simulink model "GaitAlgorithm_arduino_V3_2023a"  (R2023a)
settings: Solver=FixedStepAuto  StartTime=0.0  StopTime=inf  RelTol=1e-3  EnableMultiTasking=on
undefined symbols (not defined in the file): DiscIntNeverNeededParam, f
libraries: simulink x16, mcp2515lib x13, matrix_library x6, arduinosensorlib x4, eeGeneralControl x4, arduinolib x2, instrumentlib x2
(part 2 of 2)

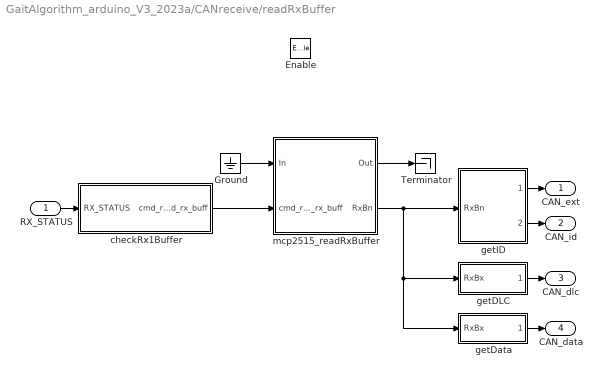
== system GaitAlgorithm_arduino_V3_2023a/CANreceive/readRxBuffer ==
  RX_STATUS : Inport
  Enable : EnablePort
  Ground : Ground
  Terminator : Terminator
  checkRx1Buffer : Subsystem  TreatAsAtomicUnit=on
  getDLC : Subsystem  TreatAsAtomicUnit=on
  getData : Subsystem  TreatAsAtomicUnit=on
  getID : Subsystem  TreatAsAtomicUnit=on
      settings: RTWSystemCode=Inline
  mcp2515_readRxBuffer : Subsystem  TreatAsAtomicUnit=on
  CAN_ext : Outport
  CAN_id : Outport  Port=2
  CAN_dlc : Outport  Port=3
  CAN_data : Outport  Port=4
  wires:
  getData/1(CAN_data) -> CAN_data/1
  mcp2515_readRxBuffer/2(RxBn) -> getID/1(RxBn), getData/1(RxBx), getDLC/1(RxBx)
  getID/2(CAN_id) -> CAN_id/1
  getID/1(CAN_ext) -> CAN_ext/1
  getDLC/1(CAN_dlc) -> CAN_dlc/1
  mcp2515_readRxBuffer/1(Out) -> Terminator/1
  Ground/1 -> mcp2515_readRxBuffer/1(In)
  RX_STATUS/1 -> checkRx1Buffer/1(RX_STATUS)
  checkRx1Buffer/1(cmd_read_rx_buff) -> mcp2515_readRxBuffer/2(cmd_read_rx_buff)

== system GaitAlgorithm_arduino_V3_2023a/CANtransmit/check TxB0 ==
  In1 : Inport
  Bitmask_TxReq : simulink/Logic and Bit Operations/Bitwise Operator  logicop=AND  UseBitMask=on  BitMask=bin2dec('00001000')  BitMaskRealWorld=Stored Integer
  CAN_FAIL : Constant  Value=2  OutDataTypeStr=int8
  CAN_OK : Constant  OutDataTypeStr=int8
  MCP_TxB0CTRL1 : Constant  Value=hex2dec('30')  OutDataTypeStr=uint8
  Switch : Switch  Criteria=u2 > Threshold  SaturateOnIntegerOverflow=off  InputSameDT=off
  mcp2515_readRegister : Subsystem  TreatAsAtomicUnit=on
  Out1 : Outport
  CANTx_Transmit : Outport  Port=2
  wires:
  CAN_FAIL/1 -> Switch/3
  mcp2515_readRegister/1(Out) -> Out1/1
  mcp2515_readRegister/2(SPI_data) -> Bitmask_TxReq/1
  MCP_TxB0CTRL1/1 -> mcp2515_readRegister/2(address)
  Bitmask_TxReq/1 -> Switch/2
  Switch/1 -> CANTx_Transmit/1
  CAN_OK/1 -> Switch/1
  In1/1 -> mcp2515_readRegister/1(In)

== system GaitAlgorithm_arduino_V3_2023a/CANtransmit/load Tx data ==
  In1 : Inport
  CAN_ext : Inport  Port=2
  CAN_id : Inport  Port=3
  CAN_dlc : Inport  Port=4
  CAN_data : Inport  Port=5
  MCP_load_TxB0 : Constant  Value=hex2dec('40')  OutDataTypeStr=uint8
  Vector Concatenate : Concatenate  NumInputs=3
  mcp2515_writeTxBuffer : Subsystem  TreatAsAtomicUnit=on
  setID : Subsystem  TreatAsAtomicUnit=on
      settings: RTWSystemCode=Inline
  Out1 : Outport
  wires:
  CAN_ext/1 -> setID/1(ext)
  CAN_id/1 -> setID/2(id)
  CAN_data/1 -> Vector Concatenate/3
  CAN_dlc/1 -> Vector Concatenate/2
  setID/1(TxBn_ID) -> Vector Concatenate/1
  In1/1 -> mcp2515_writeTxBuffer/1(In)
  mcp2515_writeTxBuffer/1(Out) -> Out1/1
  MCP_load_TxB0/1 -> mcp2515_writeTxBuffer/2(cmd_load_tx_buff)
  Vector Concatenate/1 -> mcp2515_writeTxBuffer/3(data_tx_buff)

== system GaitAlgorithm_arduino_V3_2023a/CANtransmit/send TxB0 ==
  In1 : Inport
  MCP_TxB0CTRL : Constant  Value=hex2dec('30')  OutDataTypeStr=uint8
  TxREQ : Constant  Value=8  OutDataTypeStr=uint8
  mcp2515_writeRegister : Subsystem  TreatAsAtomicUnit=on
  Out1 : Outport
  wires:
  MCP_TxB0CTRL/1 -> mcp2515_writeRegister/2(address)
  mcp2515_writeRegister/1(Out) -> Out1/1
  In1/1 -> mcp2515_writeRegister/1(In)
  TxREQ/1 -> mcp2515_writeRegister/3(value)

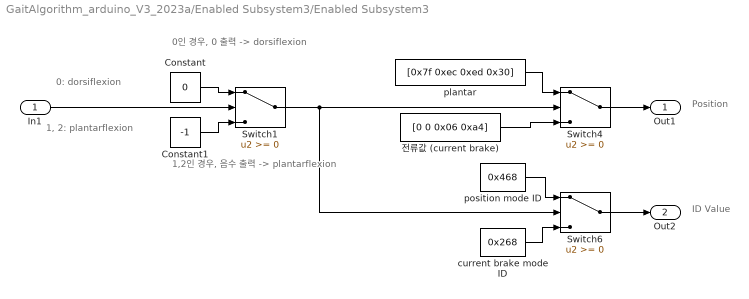
== system GaitAlgorithm_arduino_V3_2023a/Enabled Subsystem3/Enabled Subsystem3 ==
  note: ID Value
  note: Position
  note: 1,2인 경우, 음수 출력 -> plantarflexion
  note: 0인 경우, 0 출력 -> dorsiflexion
  note: 1, 2: plantarflexion
  note: 0: dorsiflexion
  In1 : Inport
  Constant : Constant  Value=0
  Constant1 : Constant  Value=-1
  Switch1 : Switch  SaturateOnIntegerOverflow=off  InputSameDT=off
  Switch4 : Switch  OutDataTypeStr=uint32  SaturateOnIntegerOverflow=off  InputSameDT=off
  Switch6 : Switch  OutDataTypeStr=uint32  SaturateOnIntegerOverflow=off  InputSameDT=off
  current brake mode ID : Constant  Value=0x268
  plantar : Constant  Value=[0x7f 0xec 0xed 0x30]
  position mode ID : Constant  Value=0x468
  전류값 (current brake) : Constant  Value=[0 0 0x06 0xa4]  OutDataTypeStr=uint8
  Out1 : Outport
  Out2 : Outport  Port=2
  wires:
  Switch6/1 -> Out2/1
  plantar/1 -> Switch4/1
  전류값 (current brake)/1 -> Switch4/3
  position mode ID/1 -> Switch6/1
  current brake mode ID/1 -> Switch6/3
  Switch4/1 -> Out1/1
  In1/1 -> Switch1/2
  Constant/1 -> Switch1/1
  Constant1/1 -> Switch1/3
  Switch1/1 -> Switch6/2, Switch4/2

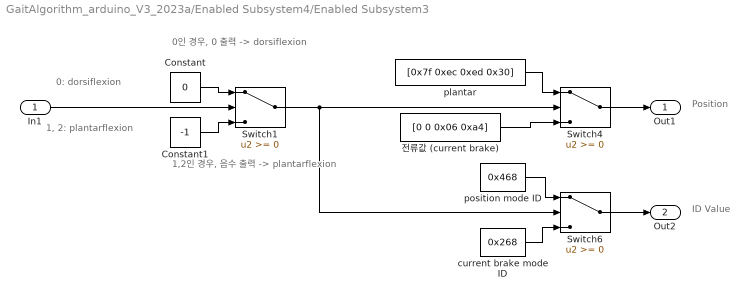
== system GaitAlgorithm_arduino_V3_2023a/Enabled Subsystem4/Enabled Subsystem3 ==
  note: ID Value
  note: Position
  note: 1,2인 경우, 음수 출력 -> plantarflexion
  note: 0인 경우, 0 출력 -> dorsiflexion
  note: 1, 2: plantarflexion
  note: 0: dorsiflexion
  In1 : Inport
  Constant : Constant  Value=0
  Constant1 : Constant  Value=-1
  Switch1 : Switch  SaturateOnIntegerOverflow=off  InputSameDT=off
  Switch4 : Switch  OutDataTypeStr=uint32  SaturateOnIntegerOverflow=off  InputSameDT=off
  Switch6 : Switch  OutDataTypeStr=uint32  SaturateOnIntegerOverflow=off  InputSameDT=off
  current brake mode ID : Constant  Value=0x268
  plantar : Constant  Value=[0x7f 0xec 0xed 0x30]
  position mode ID : Constant  Value=0x468
  전류값 (current brake) : Constant  Value=[0 0 0x06 0xa4]  OutDataTypeStr=uint8
  Out1 : Outport
  Out2 : Outport  Port=2
  wires:
  Switch6/1 -> Out2/1
  plantar/1 -> Switch4/1
  전류값 (current brake)/1 -> Switch4/3
  position mode ID/1 -> Switch6/1
  current brake mode ID/1 -> Switch6/3
  Switch4/1 -> Out1/1
  In1/1 -> Switch1/2
  Constant/1 -> Switch1/1
  Constant1/1 -> Switch1/3
  Switch1/1 -> Switch6/2, Switch4/2

== system GaitAlgorithm_arduino_V3_2023a/CANbegin/setup/changeCANmode(config) ==
  In : Inport
  MCP_CANCTRL : Constant  Value=hex2dec('0F')  OutDataTypeStr=uint8
  MODE_CONFIG : Constant  Value=hex2dec('80')  OutDataTypeStr=uint8
  MODE_MASK : Constant  Value=hex2dec('E0')  OutDataTypeStr=uint8
  mcp2515_modifyRegister : Subsystem  TreatAsAtomicUnit=on
  Out : Outport
  wires:
  MODE_CONFIG/1 -> mcp2515_modifyRegister/4(data)
  MODE_MASK/1 -> mcp2515_modifyRegister/3(mask)
  MCP_CANCTRL/1 -> mcp2515_modifyRegister/2(address)
  In/1 -> mcp2515_modifyRegister/1(In)
  mcp2515_modifyRegister/1(Out) -> Out/1

== system GaitAlgorithm_arduino_V3_2023a/CANbegin/setup/changeCANmode(normal) ==
  In : Inport
  MCP_CANCTRL : Constant  Value=hex2dec('0F')  OutDataTypeStr=uint8
  MODE_MASK : Constant  Value=hex2dec('E0')  OutDataTypeStr=uint8
  MODE_NORMAL : Constant  Value=0  OutDataTypeStr=uint8
  mcp2515_modifyRegister : Subsystem  TreatAsAtomicUnit=on
  Out : Outport
  wires:
  MODE_MASK/1 -> mcp2515_modifyRegister/3(mask)
  MODE_NORMAL/1 -> mcp2515_modifyRegister/4(data)
  MCP_CANCTRL/1 -> mcp2515_modifyRegister/2(address)
  In/1 -> mcp2515_modifyRegister/1(In)
  mcp2515_modifyRegister/1(Out) -> Out/1

== system GaitAlgorithm_arduino_V3_2023a/CANbegin/setup/mcp2515_reset ==
  In : Inport
  MCP_RESET : Constant  Value=hex2dec('C0')  OutDataTypeStr=uint8
  SPI driver : mcp2515lib/CAN application/mcp2515 driver/SPI driver  SystemSampleTime=-1  VariantActivationTime=update diagram  Latency=0  AutoFrameSizeCalculation=off
      settings: SourceProductName=CAN device driver for mcp2515
  Temporary buffer : DataStoreWrite  DataStoreName=temp_1byte  IndexOptions=Index vector (dialog)  Indices=1  OutputSizes=1
  Out : Outport
  wires:
  MCP_RESET/1 -> SPI driver/1
  In/1 -> Out/1
  SPI driver/1 -> Temporary buffer/1

== system GaitAlgorithm_arduino_V3_2023a/CANbegin/setup/setCANRxBuffer ==
  note: RXB0
  note: RXB1
  note: no filter, no mask
  In : Inport
  MCP_RXB0CTRL : Constant  Value=hex2dec('60')  OutDataTypeStr=uint8
  MCP_RXB1CTRL : Constant  Value=hex2dec('70')  OutDataTypeStr=uint8
  MCP_RXB_RX_MASK : Constant  Value=hex2dec('60')  OutDataTypeStr=uint8
  mcp2515_writeRegister : Subsystem  TreatAsAtomicUnit=on
  mcp2515_writeRegister1 : Subsystem  TreatAsAtomicUnit=on
  Out : Outport
  wires:
  MCP_RXB0CTRL/1 -> mcp2515_writeRegister/2(address)
  MCP_RXB1CTRL/1 -> mcp2515_writeRegister1/2(address)
  MCP_RXB_RX_MASK/1 -> mcp2515_writeRegister1/3(value), mcp2515_writeRegister/3(value)
  In/1 -> mcp2515_writeRegister/1(In)
  mcp2515_writeRegister1/1(Out) -> Out/1
  mcp2515_writeRegister/1(Out) -> mcp2515_writeRegister1/1(In)

== system GaitAlgorithm_arduino_V3_2023a/CANbegin/setup/setCANspeed ==
  In : Inport
  CNF1 : Inport  Port=2
  CNF2 : Inport  Port=3
  CNF3 : Inport  Port=4
  MCP_CNF1 : Constant  Value=hex2dec('2A')  OutDataTypeStr=uint8
  MCP_CNF2 : Constant  Value=hex2dec('29')  OutDataTypeStr=uint8
  MCP_CNF3 : Constant  Value=hex2dec('28')  OutDataTypeStr=uint8
  mcp2515_writeRegister1 : Subsystem  TreatAsAtomicUnit=on
  mcp2515_writeRegister2 : Subsystem  TreatAsAtomicUnit=on
  mcp2515_writeRegister3 : Subsystem  TreatAsAtomicUnit=on
  Out : Outport
  wires:
  MCP_CNF2/1 -> mcp2515_writeRegister2/2(address)
  MCP_CNF3/1 -> mcp2515_writeRegister3/2(address)
  CNF3/1 -> mcp2515_writeRegister3/3(value)
  CNF1/1 -> mcp2515_writeRegister1/3(value)
  MCP_CNF1/1 -> mcp2515_writeRegister1/2(address)
  CNF2/1 -> mcp2515_writeRegister2/3(value)
  In/1 -> mcp2515_writeRegister1/1(In)
  mcp2515_writeRegister1/1(Out) -> mcp2515_writeRegister2/1(In)
  mcp2515_writeRegister2/1(Out) -> mcp2515_writeRegister3/1(In)
  mcp2515_writeRegister3/1(Out) -> Out/1

== system GaitAlgorithm_arduino_V3_2023a/CANreceive/readRxBuffer/checkRx1Buffer ==
  RX_STATUS : Inport
  Bitmask_RxB1_Status : simulink/Logic and Bit Operations/Bitwise Operator  logicop=AND  UseBitMask=on  BitMask=bin2dec('10000000')  BitMaskRealWorld=Stored Integer
  MCP_READ_RxB0 : Constant  Value=hex2dec('90')  OutDataTypeStr=uint8
  MCP_READ_RxB1 : Constant  Value=hex2dec('94')  OutDataTypeStr=uint8
  Switch : Switch  Criteria=u2 > Threshold  SaturateOnIntegerOverflow=off  InputSameDT=off
  cmd_read_rx_buff : Outport
  wires:
  Switch/1 -> cmd_read_rx_buff/1
  MCP_READ_RxB1/1 -> Switch/1
  MCP_READ_RxB0/1 -> Switch/3
  Bitmask_RxB1_Status/1 -> Switch/2
  RX_STATUS/1 -> Bitmask_RxB1_Status/1

== system GaitAlgorithm_arduino_V3_2023a/CANreceive/readRxBuffer/getDLC ==
  RxBx : Inport
  Bitwise Operator : simulink/Logic and Bit Operations/Bitwise Operator  logicop=AND  UseBitMask=off  NumInputPorts=2  BitMask=bin2dec('11011001')  BitMaskRealWorld=Stored Integer
  MCP_DLC_MASK : Constant  Value=hex2dec('0F')  OutDataTypeStr=uint8
  RxDLC : Selector  IndexMode=Zero-based  InputPortWidth=13  IndexOptions=Index vector (dialog)  Indices=4  OutputSizes=1
  CAN_dlc : Outport
  wires:
  Bitwise Operator/1 -> CAN_dlc/1
  RxBx/1 -> RxDLC/1
  RxDLC/1 -> Bitwise Operator/1
  MCP_DLC_MASK/1 -> Bitwise Operator/2

== system GaitAlgorithm_arduino_V3_2023a/CANreceive/readRxBuffer/getData ==
  RxBx : Inport
  RxData : Selector  IndexMode=Zero-based  InputPortWidth=13  IndexOptions=Index vector (dialog)  Indices=[5:12]  OutputSizes=1
  CAN_data : Outport
  wires:
  RxBx/1 -> RxData/1
  RxData/1 -> CAN_data/1

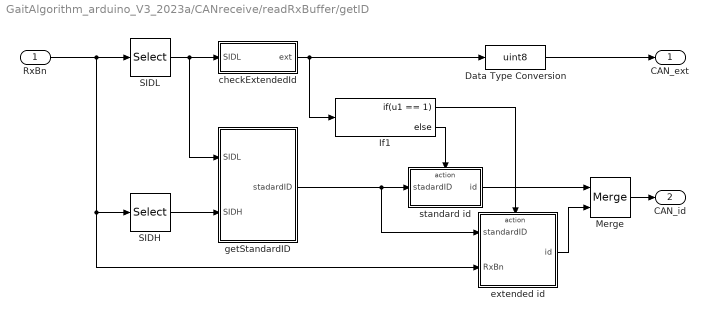
== system GaitAlgorithm_arduino_V3_2023a/CANreceive/readRxBuffer/getID ==
  RxBn : Inport
  Data Type Conversion : DataTypeConversion  OutDataTypeStr=uint8  RndMeth=Simplest  SaturateOnIntegerOverflow=off
  If1 : If  IfExpression=u1 == 1
  Merge : Merge
  SIDH : Selector  IndexMode=Zero-based  InputPortWidth=13  IndexOptions=Index vector (dialog)  Indices=0  OutputSizes=1
  SIDL : Selector  IndexMode=Zero-based  InputPortWidth=13  IndexOptions=Index vector (dialog)  Indices=1  OutputSizes=1
  checkExtendedId : Subsystem
  extended id : Subsystem  TreatAsAtomicUnit=on
      settings: RTWSystemCode=Inline
  getStandardID : Subsystem
  standard id : Subsystem  TreatAsAtomicUnit=on
      settings: RTWSystemCode=Inline
  CAN_ext : Outport
  CAN_id : Outport  Port=2
  wires:
  standard id/1(id) -> Merge/1
  extended id/1(id) -> Merge/2
  Merge/1 -> CAN_id/1
  If1/2 -> standard id/Action
  If1/1 -> extended id/Action
  RxBn/1 -> extended id/2(RxBn), SIDH/1, SIDL/1
  getStandardID/1(stadardID) -> standard id/1(stadardID), extended id/1(standardID)
  SIDL/1 -> getStandardID/1(SIDL), checkExtendedId/1(SIDL)
  SIDH/1 -> getStandardID/2(SIDH)
  checkExtendedId/1(ext) -> Data Type Conversion/1, If1/1
  Data Type Conversion/1 -> CAN_ext/1

== system GaitAlgorithm_arduino_V3_2023a/CANreceive/readRxBuffer/mcp2515_readRxBuffer ==
  In : Inport
  cmd_read_rx_buff : Inport  Port=2
  Constant : Constant  Value=zeros(1,13)  OutDataTypeStr=uint8
  SPI driver : mcp2515lib/CAN application/mcp2515 driver/SPI driver  SystemSampleTime=-1  VariantActivationTime=update diagram  Latency=0  AutoFrameSizeCalculation=off
      settings: SourceProductName=CAN device driver for mcp2515
  Selector1 : Selector  IndexMode=Zero-based  InputPortWidth=14  IndexOptions=Index vector (dialog)  Indices=[1:13]  OutputSizes=1
  Vector Concatenate : Concatenate
  Out : Outport
  RxBn : Outport  Port=2
  wires:
  cmd_read_rx_buff/1 -> Vector Concatenate/1
  Constant/1 -> Vector Concatenate/2
  Vector Concatenate/1 -> SPI driver/1
  SPI driver/1 -> Selector1/1
  Selector1/1 -> RxBn/1
  In/1 -> Out/1

== system GaitAlgorithm_arduino_V3_2023a/CANtransmit/check TxB0/mcp2515_readRegister ==
  In : Inport
  address : Inport  Port=2  OutDataTypeStr=uint8
  Constant : Constant  Value=0  OutDataTypeStr=uint8
  MCP_READ : Constant  Value=3  OutDataTypeStr=uint8
  SPI driver : mcp2515lib/CAN application/mcp2515 driver/SPI driver  SystemSampleTime=-1  VariantActivationTime=update diagram  Latency=0  AutoFrameSizeCalculation=off
      settings: SourceProductName=CAN device driver for mcp2515
  Selector : Selector  IndexMode=Zero-based  InputPortWidth=3  IndexOptions=Index vector (dialog)  Indices=2  OutputSizes=1
  Vector Concatenate : Concatenate  NumInputs=3
  Out : Outport
  SPI_data : Outport  Port=2
  wires:
  SPI driver/1 -> Selector/1
  address/1 -> Vector Concatenate/2
  Constant/1 -> Vector Concatenate/3
  In/1 -> Out/1
  MCP_READ/1 -> Vector Concatenate/1
  Selector/1 -> SPI_data/1
  Vector Concatenate/1 -> SPI driver/1

== system GaitAlgorithm_arduino_V3_2023a/CANtransmit/load Tx data/mcp2515_writeTxBuffer ==
  In : Inport
  cmd_load_tx_buff : Inport  Port=2
  data_tx_buff : Inport  Port=3
  SPI driver : mcp2515lib/CAN application/mcp2515 driver/SPI driver  SystemSampleTime=-1  VariantActivationTime=update diagram  Latency=0  AutoFrameSizeCalculation=off
      settings: SourceProductName=CAN device driver for mcp2515
  Selector1 : Selector  IndexMode=Zero-based  InputPortWidth=14  IndexOptions=Index vector (dialog)  Indices=0  OutputSizes=1
  Temporary buffer : DataStoreWrite  DataStoreName=temp_1byte  IndexOptions=Index vector (dialog)  Indices=1  OutputSizes=1
  Vector Concatenate : Concatenate
  Out : Outport
  wires:
  In/1 -> Out/1
  SPI driver/1 -> Selector1/1
  data_tx_buff/1 -> Vector Concatenate/2
  cmd_load_tx_buff/1 -> Vector Concatenate/1
  Selector1/1 -> Temporary buffer/1
  Vector Concatenate/1 -> SPI driver/1

== system GaitAlgorithm_arduino_V3_2023a/CANtransmit/load Tx data/setID ==
  ext : Inport
  id : Inport  Port=2
  Extended ID : Subsystem  TreatAsAtomicUnit=on
  If : If
  Merge : Merge
  Standard ID : Subsystem  TreatAsAtomicUnit=on
  TxBn_ID : Outport
  wires:
  ext/1 -> If/1
  If/1 -> Extended ID/Action
  If/2 -> Standard ID/Action
  Extended ID/1(TxBn_ID) -> Merge/2
  Standard ID/1(TxBn_ID) -> Merge/1
  Merge/1 -> TxBn_ID/1
  id/1 -> Extended ID/1(id), Standard ID/1(id)

== system GaitAlgorithm_arduino_V3_2023a/CANtransmit/send TxB0/mcp2515_writeRegister ==
  In : Inport
  address : Inport  Port=2  OutDataTypeStr=uint8
  value : Inport  Port=3  OutDataTypeStr=uint8
  MCP_WRITE : Constant  Value=2  OutDataTypeStr=uint8
  SPI driver : mcp2515lib/CAN application/mcp2515 driver/SPI driver  SystemSampleTime=-1  VariantActivationTime=update diagram  Latency=0  AutoFrameSizeCalculation=off
      settings: SourceProductName=CAN device driver for mcp2515
  Selector : Selector  IndexMode=Zero-based  InputPortWidth=3  IndexOptions=Index vector (dialog)  Indices=0  OutputSizes=1
  Temporary buffer : DataStoreWrite  DataStoreName=temp_1byte  IndexOptions=Index vector (dialog)  Indices=1  OutputSizes=1
  Vector Concatenate : Concatenate  NumInputs=3
  Out : Outport
  wires:
  SPI driver/1 -> Selector/1
  Selector/1 -> Temporary buffer/1
  In/1 -> Out/1
  Vector Concatenate/1 -> SPI driver/1
  value/1 -> Vector Concatenate/3
  address/1 -> Vector Concatenate/2
  MCP_WRITE/1 -> Vector Concatenate/1

== system GaitAlgorithm_arduino_V3_2023a/CANbegin/setup/changeCANmode(config)/mcp2515_modifyRegister ==
  In : Inport
  address : Inport  Port=2
  mask : Inport  Port=3
  data : Inport  Port=4
  MCP_BITMOD : Constant  Value=5  OutDataTypeStr=uint8
  SPI driver : mcp2515lib/CAN application/mcp2515 driver/SPI driver  SystemSampleTime=-1  VariantActivationTime=update diagram  Latency=0  AutoFrameSizeCalculation=off
      settings: SourceProductName=CAN device driver for mcp2515
  Selector : Selector  IndexMode=Zero-based  InputPortWidth=4  IndexOptions=Index vector (dialog)  Indices=0  OutputSizes=1
  Temporary buffer : DataStoreWrite  DataStoreName=temp_1byte  IndexOptions=Index vector (dialog)  Indices=1  OutputSizes=1
  Vector Concatenate : Concatenate  NumInputs=4
  Out : Outport
  wires:
  SPI driver/1 -> Selector/1
  data/1 -> Vector Concatenate/4
  address/1 -> Vector Concatenate/2
  mask/1 -> Vector Concatenate/3
  MCP_BITMOD/1 -> Vector Concatenate/1
  In/1 -> Out/1
  Selector/1 -> Temporary buffer/1
  Vector Concatenate/1 -> SPI driver/1

== system GaitAlgorithm_arduino_V3_2023a/CANbegin/setup/changeCANmode(normal)/mcp2515_modifyRegister ==
  In : Inport
  address : Inport  Port=2
  mask : Inport  Port=3
  data : Inport  Port=4
  MCP_BITMOD : Constant  Value=5  OutDataTypeStr=uint8
  SPI driver : mcp2515lib/CAN application/mcp2515 driver/SPI driver  SystemSampleTime=-1  VariantActivationTime=update diagram  Latency=0  AutoFrameSizeCalculation=off
      settings: SourceProductName=CAN device driver for mcp2515
  Selector : Selector  IndexMode=Zero-based  InputPortWidth=4  IndexOptions=Index vector (dialog)  Indices=0  OutputSizes=1
  Temporary buffer : DataStoreWrite  DataStoreName=temp_1byte  IndexOptions=Index vector (dialog)  Indices=1  OutputSizes=1
  Vector Concatenate : Concatenate  NumInputs=4
  Out : Outport
  wires:
  SPI driver/1 -> Selector/1
  data/1 -> Vector Concatenate/4
  address/1 -> Vector Concatenate/2
  mask/1 -> Vector Concatenate/3
  MCP_BITMOD/1 -> Vector Concatenate/1
  In/1 -> Out/1
  Selector/1 -> Temporary buffer/1
  Vector Concatenate/1 -> SPI driver/1

== system GaitAlgorithm_arduino_V3_2023a/CANbegin/setup/setCANRxBuffer/mcp2515_writeRegister ==
  In : Inport
  address : Inport  Port=2  OutDataTypeStr=uint8
  value : Inport  Port=3  OutDataTypeStr=uint8
  MCP_WRITE : Constant  Value=2  OutDataTypeStr=uint8
  SPI driver : mcp2515lib/CAN application/mcp2515 driver/SPI driver  SystemSampleTime=-1  VariantActivationTime=update diagram  Latency=0  AutoFrameSizeCalculation=off
      settings: SourceProductName=CAN device driver for mcp2515
  Selector : Selector  IndexMode=Zero-based  InputPortWidth=3  IndexOptions=Index vector (dialog)  Indices=0  OutputSizes=1
  Temporary buffer : DataStoreWrite  DataStoreName=temp_1byte  IndexOptions=Index vector (dialog)  Indices=1  OutputSizes=1
  Vector Concatenate : Concatenate  NumInputs=3
  Out : Outport
  wires:
  SPI driver/1 -> Selector/1
  Selector/1 -> Temporary buffer/1
  In/1 -> Out/1
  Vector Concatenate/1 -> SPI driver/1
  value/1 -> Vector Concatenate/3
  address/1 -> Vector Concatenate/2
  MCP_WRITE/1 -> Vector Concatenate/1

== system GaitAlgorithm_arduino_V3_2023a/CANbegin/setup/setCANRxBuffer/mcp2515_writeRegister1 ==
  In : Inport
  address : Inport  Port=2  OutDataTypeStr=uint8
  value : Inport  Port=3  OutDataTypeStr=uint8
  MCP_WRITE : Constant  Value=2  OutDataTypeStr=uint8
  SPI driver : mcp2515lib/CAN application/mcp2515 driver/SPI driver  SystemSampleTime=-1  VariantActivationTime=update diagram  Latency=0  AutoFrameSizeCalculation=off
      settings: SourceProductName=CAN device driver for mcp2515
  Selector : Selector  IndexMode=Zero-based  InputPortWidth=3  IndexOptions=Index vector (dialog)  Indices=0  OutputSizes=1
  Temporary buffer : DataStoreWrite  DataStoreName=temp_1byte  IndexOptions=Index vector (dialog)  Indices=1  OutputSizes=1
  Vector Concatenate : Concatenate  NumInputs=3
  Out : Outport
  wires:
  SPI driver/1 -> Selector/1
  Selector/1 -> Temporary buffer/1
  In/1 -> Out/1
  Vector Concatenate/1 -> SPI driver/1
  value/1 -> Vector Concatenate/3
  address/1 -> Vector Concatenate/2
  MCP_WRITE/1 -> Vector Concatenate/1

== system GaitAlgorithm_arduino_V3_2023a/CANbegin/setup/setCANspeed/mcp2515_writeRegister1 ==
  In : Inport
  address : Inport  Port=2  OutDataTypeStr=uint8
  value : Inport  Port=3  OutDataTypeStr=uint8
  MCP_WRITE : Constant  Value=2  OutDataTypeStr=uint8
  SPI driver : mcp2515lib/CAN application/mcp2515 driver/SPI driver  SystemSampleTime=-1  VariantActivationTime=update diagram  Latency=0  AutoFrameSizeCalculation=off
      settings: SourceProductName=CAN device driver for mcp2515
  Selector : Selector  IndexMode=Zero-based  InputPortWidth=3  IndexOptions=Index vector (dialog)  Indices=0  OutputSizes=1
  Temporary buffer : DataStoreWrite  DataStoreName=temp_1byte  IndexOptions=Index vector (dialog)  Indices=1  OutputSizes=1
  Vector Concatenate : Concatenate  NumInputs=3
  Out : Outport
  wires:
  SPI driver/1 -> Selector/1
  Selector/1 -> Temporary buffer/1
  In/1 -> Out/1
  Vector Concatenate/1 -> SPI driver/1
  value/1 -> Vector Concatenate/3
  address/1 -> Vector Concatenate/2
  MCP_WRITE/1 -> Vector Concatenate/1

== system GaitAlgorithm_arduino_V3_2023a/CANbegin/setup/setCANspeed/mcp2515_writeRegister2 ==
  In : Inport
  address : Inport  Port=2  OutDataTypeStr=uint8
  value : Inport  Port=3  OutDataTypeStr=uint8
  MCP_WRITE : Constant  Value=2  OutDataTypeStr=uint8
  SPI driver : mcp2515lib/CAN application/mcp2515 driver/SPI driver  SystemSampleTime=-1  VariantActivationTime=update diagram  Latency=0  AutoFrameSizeCalculation=off
      settings: SourceProductName=CAN device driver for mcp2515
  Selector : Selector  IndexMode=Zero-based  InputPortWidth=3  IndexOptions=Index vector (dialog)  Indices=0  OutputSizes=1
  Temporary buffer : DataStoreWrite  DataStoreName=temp_1byte  IndexOptions=Index vector (dialog)  Indices=1  OutputSizes=1
  Vector Concatenate : Concatenate  NumInputs=3
  Out : Outport
  wires:
  SPI driver/1 -> Selector/1
  Selector/1 -> Temporary buffer/1
  In/1 -> Out/1
  Vector Concatenate/1 -> SPI driver/1
  value/1 -> Vector Concatenate/3
  address/1 -> Vector Concatenate/2
  MCP_WRITE/1 -> Vector Concatenate/1

== system GaitAlgorithm_arduino_V3_2023a/CANbegin/setup/setCANspeed/mcp2515_writeRegister3 ==
  In : Inport
  address : Inport  Port=2  OutDataTypeStr=uint8
  value : Inport  Port=3  OutDataTypeStr=uint8
  MCP_WRITE : Constant  Value=2  OutDataTypeStr=uint8
  SPI driver : mcp2515lib/CAN application/mcp2515 driver/SPI driver  SystemSampleTime=-1  VariantActivationTime=update diagram  Latency=0  AutoFrameSizeCalculation=off
      settings: SourceProductName=CAN device driver for mcp2515
  Selector : Selector  IndexMode=Zero-based  InputPortWidth=3  IndexOptions=Index vector (dialog)  Indices=0  OutputSizes=1
  Temporary buffer : DataStoreWrite  DataStoreName=temp_1byte  IndexOptions=Index vector (dialog)  Indices=1  OutputSizes=1
  Vector Concatenate : Concatenate  NumInputs=3
  Out : Outport
  wires:
  SPI driver/1 -> Selector/1
  Selector/1 -> Temporary buffer/1
  In/1 -> Out/1
  Vector Concatenate/1 -> SPI driver/1
  value/1 -> Vector Concatenate/3
  address/1 -> Vector Concatenate/2
  MCP_WRITE/1 -> Vector Concatenate/1

== system GaitAlgorithm_arduino_V3_2023a/CANreceive/readRxBuffer/getID/checkExtendedId ==
  SIDL : Inport
  Bitmask_EXIDE : simulink/Logic and Bit Operations/Bitwise Operator  logicop=AND  UseBitMask=on  BitMask=bin2dec('00001000')  BitMaskRealWorld=Stored Integer
  MCP_TXB_EXIDE_M : Constant  Value=hex2dec('08')  OutDataTypeStr=uint8
  Relational Operator : RelationalOperator  Operator===  OutDataTypeStr=boolean  InputSameDT=off
  ext : Outport
  wires:
  Relational Operator/1 -> ext/1
  MCP_TXB_EXIDE_M/1 -> Relational Operator/1
  Bitmask_EXIDE/1 -> Relational Operator/2
  SIDL/1 -> Bitmask_EXIDE/1

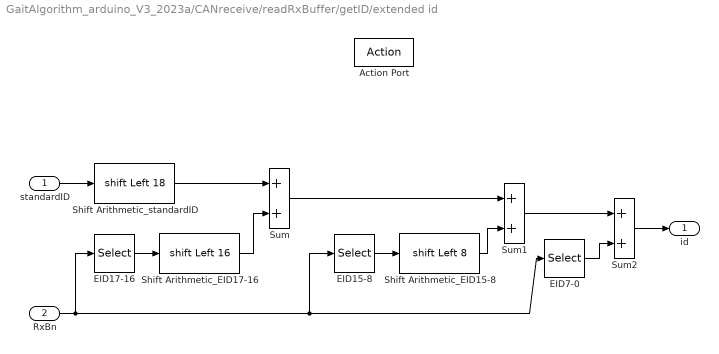
== system GaitAlgorithm_arduino_V3_2023a/CANreceive/readRxBuffer/getID/extended id ==
  standardID : Inport
  RxBn : Inport  Port=2
  Action Port : ActionPort  ActionPortLabel=if(u1 == 1)
  EID15-8 : Selector  IndexMode=Zero-based  InputPortWidth=13  IndexOptions=Index vector (dialog)  Indices=2  OutputSizes=1
  EID17-16 : Selector  IndexMode=Zero-based  InputPortWidth=13  IndexOptions=Index vector (dialog)  Indices=1  OutputSizes=1
  EID7-0 : Selector  IndexMode=Zero-based  InputPortWidth=13  IndexOptions=Index vector (dialog)  Indices=3  OutputSizes=1
  Shift Arithmetic_EID15-8 : ArithShift  BitShiftNumber=8  BitShiftDirection=Left
  Shift Arithmetic_EID17-16 : ArithShift  BitShiftNumber=16  BitShiftDirection=Left
  Shift Arithmetic_standardID : ArithShift  BitShiftNumber=18  BitShiftDirection=Left
  Sum : Sum
  Sum1 : Sum
  Sum2 : Sum
  id : Outport
  wires:
  Sum2/1 -> id/1
  standardID/1 -> Shift Arithmetic_standardID/1
  Shift Arithmetic_standardID/1 -> Sum/1
  EID17-16/1 -> Shift Arithmetic_EID17-16/1
  Shift Arithmetic_EID17-16/1 -> Sum/2
  Sum/1 -> Sum1/1
  Shift Arithmetic_EID15-8/1 -> Sum1/2
  EID15-8/1 -> Shift Arithmetic_EID15-8/1
  Sum1/1 -> Sum2/1
  RxBn/1 -> EID7-0/1, EID15-8/1, EID17-16/1
  EID7-0/1 -> Sum2/2

== system GaitAlgorithm_arduino_V3_2023a/CANreceive/readRxBuffer/getID/getStandardID ==
  SIDL : Inport
  SIDH : Inport  Port=2
  Bitmask_SID2-0 : simulink/Logic and Bit Operations/Bitwise Operator  logicop=AND  UseBitMask=on  BitMask=bin2dec('11100000')  BitMaskRealWorld=Stored Integer
  Data Type Conversion : DataTypeConversion  OutDataTypeStr=uint32  SaturateOnIntegerOverflow=off  RndMeth=Floor
  Shift Arithmetic_SID10-3 : ArithShift  BitShiftNumber=3  BitShiftDirection=Left
  Shift Arithmetic_SID2-0 : ArithShift  BitShiftNumber=5  BitShiftDirection=Right
  Sum1 : Sum
  stadardID : Outport
  wires:
  Sum1/1 -> stadardID/1
  Shift Arithmetic_SID2-0/1 -> Sum1/1
  Shift Arithmetic_SID10-3/1 -> Sum1/2
  SIDL/1 -> Bitmask_SID2-0/1
  SIDH/1 -> Data Type Conversion/1
  Bitmask_SID2-0/1 -> Shift Arithmetic_SID2-0/1
  Data Type Conversion/1 -> Shift Arithmetic_SID10-3/1

== system GaitAlgorithm_arduino_V3_2023a/CANreceive/readRxBuffer/getID/standard id ==
  stadardID : Inport
  Action Port : ActionPort  ActionPortLabel=else
  id : Outport
  wires:
  stadardID/1 -> id/1

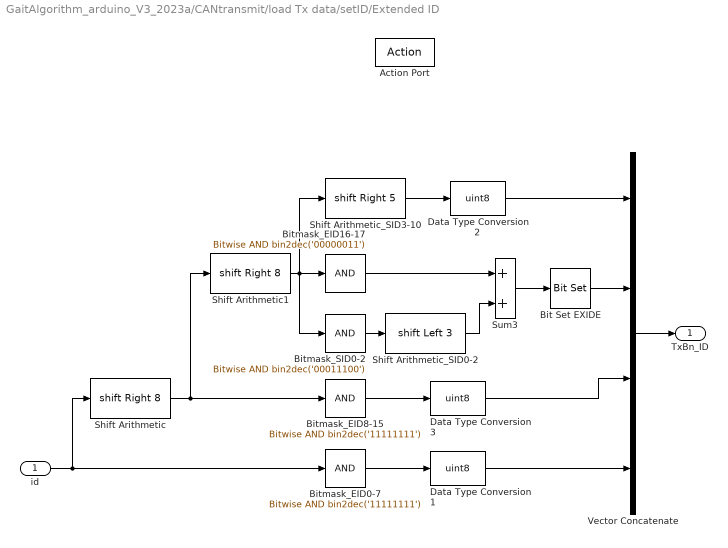
== system GaitAlgorithm_arduino_V3_2023a/CANtransmit/load Tx data/setID/Extended ID ==
  id : Inport
  Action Port : ActionPort  ActionPortLabel=if(u1 > 0)
  Bit Set EXIDE : simulink/Logic and Bit Operations/Bit Set  iBit=3
  Bitmask_EID0-7 : simulink/Logic and Bit Operations/Bitwise Operator  logicop=AND  UseBitMask=on  BitMask=bin2dec('11111111')  BitMaskRealWorld=Stored Integer
  Bitmask_EID16-17 : simulink/Logic and Bit Operations/Bitwise Operator  logicop=AND  UseBitMask=on  BitMask=bin2dec('00000011')  BitMaskRealWorld=Stored Integer
  Bitmask_EID8-15 : simulink/Logic and Bit Operations/Bitwise Operator  logicop=AND  UseBitMask=on  BitMask=bin2dec('11111111')  BitMaskRealWorld=Stored Integer
  Bitmask_SID0-2 : simulink/Logic and Bit Operations/Bitwise Operator  logicop=AND  UseBitMask=on  BitMask=bin2dec('00011100')  BitMaskRealWorld=Stored Integer
  Data Type Conversion1 : DataTypeConversion  OutDataTypeStr=uint8  RndMeth=Simplest  SaturateOnIntegerOverflow=off
  Data Type Conversion2 : DataTypeConversion  OutDataTypeStr=uint8  RndMeth=Simplest  SaturateOnIntegerOverflow=off
  Data Type Conversion3 : DataTypeConversion  OutDataTypeStr=uint8  RndMeth=Simplest  SaturateOnIntegerOverflow=off
  Shift Arithmetic : ArithShift  BitShiftNumber=8  BitShiftDirection=Right
  Shift Arithmetic1 : ArithShift  BitShiftNumber=8  BitShiftDirection=Right
  Shift Arithmetic_SID0-2 : ArithShift  BitShiftNumber=3  BitShiftDirection=Left
  Shift Arithmetic_SID3-10 : ArithShift  BitShiftNumber=5  BitShiftDirection=Right
  Sum3 : Sum  OutDataTypeStr=uint8
  Vector Concatenate : Concatenate  NumInputs=4
  TxBn_ID : Outport
  wires:
  Vector Concatenate/1 -> TxBn_ID/1
  id/1 -> Shift Arithmetic/1, Bitmask_EID0-7/1
  Bitmask_EID0-7/1 -> Data Type Conversion1/1
  Data Type Conversion1/1 -> Vector Concatenate/4
  Shift Arithmetic/1 -> Shift Arithmetic1/1, Bitmask_EID8-15/1
  Bitmask_EID8-15/1 -> Data Type Conversion3/1
  Data Type Conversion3/1 -> Vector Concatenate/3
  Shift Arithmetic1/1 -> Shift Arithmetic_SID3-10/1, Bitmask_SID0-2/1, Bitmask_EID16-17/1
  Sum3/1 -> Bit Set EXIDE/1
  Bitmask_EID16-17/1 -> Sum3/1
  Bitmask_SID0-2/1 -> Shift Arithmetic_SID0-2/1
  Shift Arithmetic_SID0-2/1 -> Sum3/2
  Bit Set EXIDE/1 -> Vector Concatenate/2
  Shift Arithmetic_SID3-10/1 -> Data Type Conversion2/1
  Data Type Conversion2/1 -> Vector Concatenate/1

== system GaitAlgorithm_arduino_V3_2023a/CANtransmit/load Tx data/setID/Standard ID ==
  id : Inport
  Action Port : ActionPort  ActionPortLabel=else
  Vector Concatenate : Concatenate  NumInputs=4
  convert_ID : Subsystem  TreatAsAtomicUnit=on
  no data : Constant  Value=0  OutDataTypeStr=uint8
  TxBn_ID : Outport
  wires:
  Vector Concatenate/1 -> TxBn_ID/1
  no data/1 -> Vector Concatenate/3, Vector Concatenate/4
  convert_ID/2(SIDL) -> Vector Concatenate/2
  id/1 -> convert_ID/1(id)
  convert_ID/1(SIDH) -> Vector Concatenate/1

== system GaitAlgorithm_arduino_V3_2023a/CANtransmit/load Tx data/setID/Standard ID/convert_ID ==
  id : Inport
  Bitmask_SID0-10 : simulink/Logic and Bit Operations/Bitwise Operator  logicop=AND  UseBitMask=on  BitMask=bin2dec('0000011111111111')  BitMaskRealWorld=Stored Integer
  Bitmask_SID0-2 : simulink/Logic and Bit Operations/Bitwise Operator  logicop=AND  UseBitMask=on  BitMask=bin2dec('0000000011100000')  BitMaskRealWorld=Stored Integer
  Data Type Conversion1 : DataTypeConversion  OutDataTypeStr=uint8  RndMeth=Simplest  SaturateOnIntegerOverflow=off
  Data Type Conversion2 : DataTypeConversion  OutDataTypeStr=uint8  RndMeth=Simplest  SaturateOnIntegerOverflow=off
  Shift Arithmetic1 : ArithShift  BitShiftNumber=3  BitShiftDirection=Right
  Shift Arithmetic2 : ArithShift  BitShiftNumber=5  BitShiftDirection=Left
  SIDH : Outport
  SIDL : Outport  Port=2
  wires:
  Shift Arithmetic1/1 -> Data Type Conversion1/1
  Data Type Conversion1/1 -> SIDH/1
  Bitmask_SID0-10/1 -> Shift Arithmetic2/1, Shift Arithmetic1/1
  Data Type Conversion2/1 -> SIDL/1
  Shift Arithmetic2/1 -> Bitmask_SID0-2/1
  id/1 -> Bitmask_SID0-10/1
  Bitmask_SID0-2/1 -> Data Type Conversion2/1
